simulink model "CruiseControl_Harness_SB_StandAlone"  (R2016b)
settings: Solver=FixedStepDiscrete  StartTime=0.0  StopTime=2  FixedStep=0.1  RelTol=1e-3  EnableMultiTasking=on
undefined symbols (not defined in the file): sigbuilder_block
settings Model: Creator=colosky  LastModifiedBy=colosky
settings DataIOCC: LimitDataPoints=on  SaveFormat=Array  SaveOutput=off  SignalLogging=off  DSMLogging=off  SaveTime=off
settings OptimizationCC: DefaultParameterBehavior=Inlined  InlineInvariantSignals=on  ExpressionDepthLimit=2147483647  InitFltsAndDblsToZero=on  NoFixptDivByZeroProtection=on  LifeSpan=inf
settings DebuggingCC: SignalInfNanChecking=warning  SaveWithParameterizedLinksMsg=none  UnderspecifiedInitializationDetection=Classic  MergeDetectMultiDrivingBlocksExec=none  SolverPrmCheckMsg=warning  FcnCallInpInsideContextMsg=warning  UniqueDataStoreMsg=warning  AllowSymbolicDim=off  StateNameClashWarn=warning  StrictBusMsg=ErrorOnBusTreatedAsVector  SFUnexpectedBacktrackingDiag=warning  SFNoUnconditionalDefaultTransitionDiag=warning  SFExecutionAtInitializationDiag=none
settings HardwareCC: ProdBitPerPointer=32  ProdBitPerSizeT=32  ProdBitPerPtrDiffT=32  ProdLargestAtomicFloat=None  ProdIntDivRoundTo=Undefined  ProdEndianess=Unspecified  ProdWordSize=32  ProdHWDeviceType=32-bit Generic
settings ModelReferenceCC: ModelReferenceNumInstancesAllowed=Single  PropagateSignalLabelsOutOfModel=off
settings SFSimCC: SimParseCustomCode=off
settings RTWCC: SystemTargetFile=ert.tlc  TemplateMakefile=ert_default_tmf  Description=Embedded Coder  GenerateReport=on  IncludeHyperlinkInReport=on  LaunchReport=on  PortableWordSizes=on  GenerateTraceInfo=on  GenerateTraceReport=on  GenerateTraceReportSl=on  GenerateTraceReportSf=on  GenerateTraceReportEml=on
settings CodeAppCC: IgnoreCustomStorageClasses=off  CustomSymbolStrGlobalVar=$N$M
settings ERTTargetCC: GenerateSampleERTMain=on  InlinedParameterPlacement=NonHierarchical  ERTCustomFileTemplate=example_file_process.tlc  ConvertIfToSwitch=off  SuppressUnreachableDefaultCases=off
settings ConfigComp: CovEnable=on  CovScope=ReferencedModels  CovIncludeTopModel=off  CovMetricSettings=dcme  CovHTMLOptions=-sRT=1 -sVT=0 -aTS=1 -bRG=1 -bTC=1 -hTR=0 -nFC=0 -nFD=1 -scm=1 -bcm=1 -xEv=0 -xEM=0  CovModelRefEnable=all  CovExternalEMLEnable=off  CovSFcnEnable=off  DVMode=DesignErrorDetection  DVMaxProcessTime=3000  DVDisplayUnsatisfiableObjectives=on  DVAutomaticStubbing=off  DVMakeOutputFilesUnique=off  DVParameters=on  DVParametersUseConfig=on  DVModelCoverageObjectives=MCDC  DVMaxTestCaseSteps=500  DVTestSuiteOptimization=CombinedObjectives  DVAssertions=EnableAll  DVProofAssumptions=EnableAll  DVIgnoreCovSatisfied=on  DVCoverageDataFile=CruiseControlCovManual.cvt  DVDetectIntegerOverflow=off  DVDetectDeadLogic=on  DVDetectActiveLogic=on  DVDetectFloatOverflow=off  DVMaxViolationSteps=50  DVSaveDataFile=off  DVSaveHarnessModel=on  DVHarnessModelFileName=$ModelName$_harness_SLDV  DVReportIncludeGraphics=on  PSAutoStubLUT=off

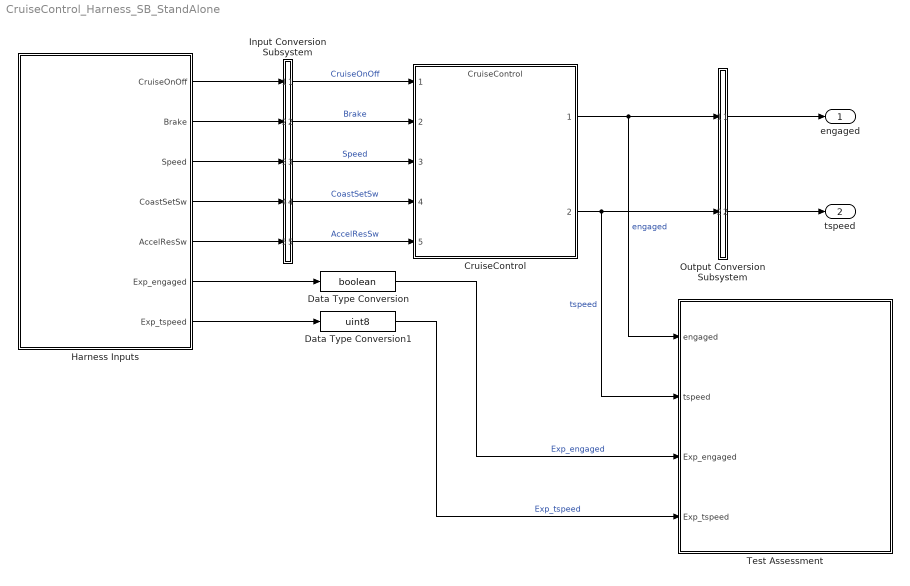
== system CruiseControl_Harness_SB_StandAlone ==
  CruiseControl : ModelReference  ModelNameDialog=CruiseControl  SimulationMode=Normal  ModelReferenceVersion=1.475
  Data Type Conversion : DataTypeConversion  OutDataTypeStr=boolean
  Data Type Conversion1 : DataTypeConversion  OutDataTypeStr=uint8
  Harness Inputs : Subsystem  Tag=STV Subsys  LoadFcn=sigbuilder_block('load',[-9.6 94.2 520.2 400.2 ]);  StartFcn=sigbuilder_block('start');  StopFcn=sigbuilder_block('stop');  ClipboardFcn=sigbuilder_block('clipboard');  mask(Sigbuilder block){tuvar=[0:10]}
      mask init:
      | if ~strcmp(get_param(bdroot(gcb),'SimulationStatus'),'stopped'),tuvar = sigbuilder_block('maskInit'); end
      settings: CopyFcn=sigbuilder_block('copy');  DeleteFcn=sigbuilder_block('delete');  ModelCloseFcn=sigbuilder_block('modelClose');  PreSaveFcn=sigbuilder_block('preSave');  PauseFcn=sigbuilder_block('pause');  ContinueFcn=sigbuilder_block('continue');  NameChangeFcn=sigbuilder_block('namechange');  OpenFcn=sigbuilder_block('open',[58.2 96 520.2 400.2 ]);  CloseFcn=sigbuilder_block('close');
      mask Display: plot(0, 0, 100, 100,[2, 2, 32, 32, 2], [68, 8, 8, 68, 68],[32, 2], [38, 38], [32, 19, 2],[53, 60, 44], [32, 17, 17, 2],[16, 16, 31, 31]);txt = getActiveGroup(gcbh);text(2, 100, txt,'verticalAlignment', 'top');
  Input Conversion Subsystem : Subsystem  Tag=_input_conv_ss_
  Output Conversion Subsystem : Subsystem  Tag=_output_conv_ss_
  Test Assessment : State Transition Table  TreatAsAtomicUnit=on
  engaged : Outport  OutDataTypeStr=boolean  PortDimensions=[1]
  tspeed : Outport  Port=2  OutDataTypeStr=uint8  PortDimensions=[1]
  wires:
  Input Conversion Subsystem/1(Out_1) -> CruiseControl/1  "CruiseOnOff"
  Input Conversion Subsystem/2(Out_2) -> CruiseControl/2  "Brake"
  Input Conversion Subsystem/3(Out_3) -> CruiseControl/3  "Speed"
  Input Conversion Subsystem/4(Out_4) -> CruiseControl/4  "CoastSetSw"
  Input Conversion Subsystem/5(Out_5) -> CruiseControl/5  "AccelResSw"
  Output Conversion Subsystem/1(Out_1) -> engaged/1
  Output Conversion Subsystem/2(Out_2) -> tspeed/1
  CruiseControl/1 -> Output Conversion Subsystem/1(In_1), Test Assessment/1(engaged)  "engaged"
  CruiseControl/2 -> Output Conversion Subsystem/2(In_2), Test Assessment/2(tspeed)  "tspeed"
  Harness Inputs/1(CruiseOnOff) -> Input Conversion Subsystem/1(In_1)
  Harness Inputs/2(Brake) -> Input Conversion Subsystem/2(In_2)
  Harness Inputs/3(Speed) -> Input Conversion Subsystem/3(In_3)
  Harness Inputs/4(CoastSetSw) -> Input Conversion Subsystem/4(In_4)
  Harness Inputs/5(AccelResSw) -> Input Conversion Subsystem/5(In_5)
  Harness Inputs/6(Exp_engaged) -> Data Type Conversion/1
  Harness Inputs/7(Exp_tspeed) -> Data Type Conversion1/1
  Data Type Conversion/1 -> Test Assessment/3(Exp_engaged)  "Exp_engaged"
  Data Type Conversion1/1 -> Test Assessment/4(Exp_tspeed)  "Exp_tspeed"

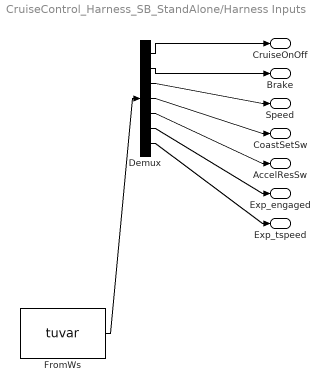
== system CruiseControl_Harness_SB_StandAlone/Harness Inputs ==
  Demux : Demux  Tag=STV Demux  Outputs=7
  FromWs : FromWorkspace  Tag=STV FromWs  VariableName=tuvar  SampleTime=0
      SigBuilderData=|
      | dataSet(1).timeRange = [0 2]
      | dataSet(1).name = 'Init Not Enable or Engaged'
      | dataSet(2).timeRange = [0 2]
      | dataSet(2).name = 'Not Engaged with Enable'
      | dataSet(3).timeRange = [0 2]
      | dataSet(3).name = 'Disengage with Disable'
      | dataSet(4).timeRange = [0 2]
      | dataSet(4).name = 'Engage 1st with CoastSetSW'
      | dataSet(5).timeRange = [0 2]
      | dataSet(5).name = 'No Engage 1st with AccelResSW'
      | dataSet(6).timeRange = [0 2]
      | dataSet(6).name = 'Disengage with Brake'
      | dataSet(7).timeRange = [0 2]
      | dataSet(7).name = 'Re-Engage with CoastSetSw'
      | dataSet(8).timeRange = [0 2]
      | dataSet(8).name = 'Re-Engage with AccelResSw'
      | dataSet(9).timeRange = [0 2]
      | dataSet(9).name = 'Engaged Decel with CoastSetSW'
      | dataSet(10).timeRange = [0 2]
      | dataSet(10).name = 'Engaged Accel with AccelResSW '
      | dataSet(11).timeRange = [0 2]
      | dataSet(11).name = 'Engagd Decel with CoastSet Hold'
      | dataSet(12).timeRange = [0 2]
      | dataSet(12).name = 'Engagd Accel with AccelRes Hold'
      | dataSet(13).timeRange = [0 2]
      | dataSet(13).name = 'Engage CoastSetSw Veh Spd'
      | dataSet(14).timeRange = [0 2]
      | dataSet(14).name = 'Engage AccelResSw Veh Spd '
      | sbobj.Name = 'Signal Builder'
      | sbobj.Groups(1).Name = 'Init Not Enable or Engaged'
      | sbobj.Groups(1).Signals(1).Name = 'CruiseOnOff'
      | sbobj.Groups(1).Signals(1).XData = [0 1 2]
      | sbobj.Groups(1).Signals(1).YData = [0 0 0]
      | sbobj.Groups(1).Signals(2).Name = 'Brake'
      | sbobj.Groups(1).Signals(2).XData = [0 1 2]
      | sbobj.Groups(1).Signals(2).YData = [0 0 0]
      | sbobj.Groups(1).Signals(3).Name = 'Speed'
      | sbobj.Groups(1).Signals(3).XData = [0 1 2]
      | sbobj.Groups(1).Signals(3).YData = [50 50 50]
      | sbobj.Groups(1).Signals(4).Name = 'CoastSetSw'
      | sbobj.Groups(1).Signals(4).XData = [0 1 2]
      | sbobj.Groups(1).Signals(4).YData = [0 0 0]
      | sbobj.Groups(1).Signals(5).Name = 'AccelResSw'
      | sbobj.Groups(1).Signals(5).XData = [0 1 2]
      | sbobj.Groups(1).Signals(5).YData = [0 0 0]
      | sbobj.Groups(1).Signals(6).Name = 'Exp_engaged'
      | sbobj.Groups(1).Signals(6).XData = [0 1 2]
      | sbobj.Groups(1).Signals(6).YData = [0 0 0]
      | sbobj.Groups(1).Signals(7).Name = 'Exp_tspeed'
      | sbobj.Groups(1).Signals(7).XData = [0 1 2]
      | sbobj.Groups(1).Signals(7).YData = [0 0 0]
      | sbobj.Groups(1).TimeRange = [0 2]
      | sbobj.Groups(2).Name = 'Not Engaged with Enable'
      | sbobj.Groups(2).Signals(1).Name = 'CruiseOnOff'
      | sbobj.Groups(2).Signals(1).XData = [0 1 1 1.5 1.5 2]
      | sbobj.Groups(2).Signals(1).YData = [0 0 1 1 0 0]
      | sbobj.Groups(2).Signals(2).Name = 'Brake'
      | sbobj.Groups(2).Signals(2).XData = [0 1 1.5 2]
      | sbobj.Groups(2).Signals(2).YData = [0 0 0 0]
      | sbobj.Groups(2).Signals(3).Name = 'Speed'
      | sbobj.Groups(2).Signals(3).XData = [0 1 1.5 2]
      | sbobj.Groups(2).Signals(3).YData = [0 0 0 0]
      | sbobj.Groups(2).Signals(4).Name = 'CoastSetSw'
      | sbobj.Groups(2).Signals(4).XData = [0 1 1.5 2]
      | sbobj.Groups(2).Signals(4).YData = [0 0 0 0]
      | sbobj.Groups(2).Signals(5).Name = 'AccelResSw'
      | sbobj.Groups(2).Signals(5).XData = [0 1 1.5 2]
      | sbobj.Groups(2).Signals(5).YData = [0 0 0 0]
      | sbobj.Groups(2).Signals(6).Name = 'Exp_engaged'
      | sbobj.Groups(2).Signals(6).XData = [0 1 1.5 2]
      | sbobj.Groups(2).Signals(6).YData = [0 0 0 0]
      | sbobj.Groups(2).Signals(7).Name = 'Exp_tspeed'
      | sbobj.Groups(2).Signals(7).XData = [0 1 1.5 2]
      | sbobj.Groups(2).Signals(7).YData = [0 0 0 0]
      | sbobj.Groups(2).TimeRange = [0 2]
      | sbobj.Groups(3).Name = 'Disengage with Disable'
      | sbobj.Groups(3).Signals(1).Name = 'CruiseOnOff'
      | sbobj.Groups(3).Signals(1).XData = [0 0.5 0.5 1 1.1 1.5 1.5 2]
      | sbobj.Groups(3).Signals(1).YData = [0 0 1 1 1 1 0 0]
      | sbobj.Groups(3).Signals(2).Name = 'Brake'
      | sbobj.Groups(3).Signals(2).XData = [0 0.5 1 1.1 1.5 2]
      | sbobj.Groups(3).Signals(2).YData = [0 0 0 0 0 0]
      | sbobj.Groups(3).Signals(3).Name = 'Speed'
      | sbobj.Groups(3).Signals(3).XData = [0 0.5 1 1.1 1.5 2]
      | sbobj.Groups(3).Signals(3).YData = [50 50 50 50 50 50]
      | sbobj.Groups(3).Signals(4).Name = 'CoastSetSw'
      | sbobj.Groups(3).Signals(4).XData = [0 0.5 1 1 1.1 1.1 1.5 2]
      | sbobj.Groups(3).Signals(4).YData = [0 0 0 1 1 0 0 0]
      | sbobj.Groups(3).Signals(5).Name = 'AccelResSw'
      | sbobj.Groups(3).Signals(5).XData = [0 0.5 1 1.1 1.5 2]
      | sbobj.Groups(3).Signals(5).YData = [0 0 0 0 0 0]
      | sbobj.Groups(3).Signals(6).Name = 'Exp_engaged'
      | sbobj.Groups(3).Signals(6).XData = [0 0.5 1 1 1.1 1.5 1.5 2]
      | sbobj.Groups(3).Signals(6).YData = [0 0 0 1 1 1 0 0]
      | sbobj.Groups(3).Signals(7).Name = 'Exp_tspeed'
      | sbobj.Groups(3).Signals(7).XData = [0 0.5 1 1 1.1 1.5 1.5 2]
      | sbobj.Groups(3).Signals(7).YData = [0 0 0 50 50 50 0 0]
      | sbobj.Groups(3).TimeRange = [0 2]
      | sbobj.Groups(4).Name = 'Engage 1st with CoastSetSW'
      | sbobj.Groups(4).Signals(1).Name = 'CruiseOnOff'
      | sbobj.Groups(4).Signals(1).XData = [0 0.5 0.5 1 1.1 2]
      | sbobj.Groups(4).Signals(1).YData = [0 0 1 1 1 1]
      | sbobj.Groups(4).Signals(2).Name = 'Brake'
      | sbobj.Groups(4).Signals(2).XData = [0 0.5 1 1.1 2]
      | sbobj.Groups(4).Signals(2).YData = [0 0 0 0 0]
      | sbobj.Groups(4).Signals(3).Name = 'Speed'
      | sbobj.Groups(4).Signals(3).XData = [0 0.5 1 1.1 2]
      | sbobj.Groups(4).Signals(3).YData = [50 50 50 50 50]
      | sbobj.Groups(4).Signals(4).Name = 'CoastSetSw'
      | sbobj.Groups(4).Signals(4).XData = [0 0.5 1 1 1.1 1.1 2]
      | sbobj.Groups(4).Signals(4).YData = [0 0 0 1 1 0 0]
      | sbobj.Groups(4).Signals(5).Name = 'AccelResSw'
      | sbobj.Groups(4).Signals(5).XData = [0 0.5 1 1.1 2]
      | sbobj.Groups(4).Signals(5).YData = [0 0 0 0 0]
      | sbobj.Groups(4).Signals(6).Name = 'Exp_engaged'
      | sbobj.Groups(4).Signals(6).XData = [0 0.5 1 1 1.1 2]
      | sbobj.Groups(4).Signals(6).YData = [0 0 0 1 1 1]
      | sbobj.Groups(4).Signals(7).Name = 'Exp_tspeed'
      | sbobj.Groups(4).Signals(7).XData = [0 0.5 1 1 1.1 2]
      | sbobj.Groups(4).Signals(7).YData = [0 0 0 50 50 50]
      | sbobj.Groups(4).TimeRange = [0 2]
      | sbobj.Groups(5).Name = 'No Engage 1st with AccelResSW'
      | sbobj.Groups(5).Signals(1).Name = 'CruiseOnOff'
      | sbobj.Groups(5).Signals(1).XData = [0 0.5 0.5 1 1.1 2]
      | sbobj.Groups(5).Signals(1).YData = [0 0 1 1 1 1]
      | sbobj.Groups(5).Signals(2).Name = 'Brake'
      | sbobj.Groups(5).Signals(2).XData = [0 0.5 1 1.1 2]
      | sbobj.Groups(5).Signals(2).YData = [0 0 0 0 0]
      | sbobj.Groups(5).Signals(3).Name = 'Speed'
      | sbobj.Groups(5).Signals(3).XData = [0 0.5 1 1.1 2]
      | sbobj.Groups(5).Signals(3).YData = [50 50 50 50 50]
      | sbobj.Groups(5).Signals(4).Name = 'CoastSetSw'
      | sbobj.Groups(5).Signals(4).XData = [0 0.5 1 1.1 2]
      | sbobj.Groups(5).Signals(4).YData = [0 0 0 0 0]
      | sbobj.Groups(5).Signals(5).Name = 'AccelResSw'
      | sbobj.Groups(5).Signals(5).XData = [0 0.5 1 1 1.1 1.1 2]
      | sbobj.Groups(5).Signals(5).YData = [0 0 0 1 1 0 0]
      | sbobj.Groups(5).Signals(6).Name = 'Exp_engaged'
      | sbobj.Groups(5).Signals(6).XData = [0 0.5 1 1.1 2]
      | sbobj.Groups(5).Signals(6).YData = [0 0 0 0 0]
      | sbobj.Groups(5).Signals(7).Name = 'Exp_tspeed'
      | sbobj.Groups(5).Signals(7).XData = [0 0.5 1 1.1 2]
      | sbobj.Groups(5).Signals(7).YData = [0 0 0 0 0]
      | sbobj.Groups(5).TimeRange = [0 2]
      | sbobj.Groups(6).Name = 'Disengage with Brake'
      | sbobj.Groups(6).Signals(1).Name = 'CruiseOnOff'
      | sbobj.Groups(6).Signals(1).XData = [0 0.5 0.5 1 1.1 1.5 1.6 2]
      | sbobj.Groups(6).Signals(1).YData = [0 0 1 1 1 1 1 1]
      | sbobj.Groups(6).Signals(2).Name = 'Brake'
      | sbobj.Groups(6).Signals(2).XData = [0 0.5 1 1.1 1.5 1.5 1.6 1.6 2]
      | sbobj.Groups(6).Signals(2).YData = [0 0 0 0 0 1 1 0 0]
      | sbobj.Groups(6).Signals(3).Name = 'Speed'
      | sbobj.Groups(6).Signals(3).XData = [0 0.5 1 1.1 1.5 1.6 2]
      | sbobj.Groups(6).Signals(3).YData = [50 50 50 50 50 50 50]
      | sbobj.Groups(6).Signals(4).Name = 'CoastSetSw'
      | sbobj.Groups(6).Signals(4).XData = [0 0.5 1 1 1.1 1.1 1.5 1.6 2]
      | sbobj.Groups(6).Signals(4).YData = [0 0 0 1 1 0 0 0 0]
      | sbobj.Groups(6).Signals(5).Name = 'AccelResSw'
      | sbobj.Groups(6).Signals(5).XData = [0 0.5 1 1.1 1.5 1.6 2]
      | sbobj.Groups(6).Signals(5).YData = [0 0 0 0 0 0 0]
      | sbobj.Groups(6).Signals(6).Name = 'Exp_engaged'
      | sbobj.Groups(6).Signals(6).XData = [0 0.5 1 1 1.1 1.5 1.5 1.6 2]
      | sbobj.Groups(6).Signals(6).YData = [0 0 0 1 1 1 0 0 0]
      | sbobj.Groups(6).Signals(7).Name = 'Exp_tspeed'
      | sbobj.Groups(6).Signals(7).XData = [0 0.5 1 1 1.1 1.5 1.6 2]
      | sbobj.Groups(6).Signals(7).YData = [0 0 0 50 50 50 50 50]
      | sbobj.Groups(6).TimeRange = [0 2]
      | sbobj.Groups(7).Name = 'Re-Engage with CoastSetSw'
      | sbobj.Groups(7).Signals(1).Name = 'CruiseOnOff'
      | sbobj.Groups(7).Signals(1).XData = [0 0.5 0.5 1 1.1 1.3 1.5 1.7 1.8 2]
      | sbobj.Groups(7).Signals(1).YData = [0 0 1 1 1 1 1 1 1 1]
      | sbobj.Groups(7).Signals(2).Name = 'Brake'
      | sbobj.Groups(7).Signals(2).XData = [0 0.5 1 1.1 1.3 1.3 1.5 1.5 1.7 1.8 2]
      | sbobj.Groups(7).Signals(2).YData = [0 0 0 0 0 1 1 0 0 0 0]
      | sbobj.Groups(7).Signals(3).Name = 'Speed'
      | sbobj.Groups(7).Signals(3).XData = [0 0.5 1 1.1 1.3 1.5 1.7 1.7 1.8 2]
      | sbobj.Groups(7).Signals(3).YData = [50 50 50 50 50 50 50 60 60 60]
      | sbobj.Groups(7).Signals(4).Name = 'CoastSetSw'
      | sbobj.Groups(7).Signals(4).XData = [0 0.5 1 1 1.1 1.1 1.3 1.5 1.7 1.7 1.8 1.8 2]
      | sbobj.Groups(7).Signals(4).YData = [0 0 0 1 1 0 0 0 0 1 1 0 0]
      | sbobj.Groups(7).Signals(5).Name = 'AccelResSw'
      | sbobj.Groups(7).Signals(5).XData = [0 0.5 1 1.1 1.3 1.5 1.7 1.8 2]
      | sbobj.Groups(7).Signals(5).YData = [0 0 0 0 0 0 0 0 0]
      | sbobj.Groups(7).Signals(6).Name = 'Exp_engaged'
      | sbobj.Groups(7).Signals(6).XData = [0 0.5 1 1 1.1 1.3 1.3 1.5 1.7 1.7 1.8 2]
      | sbobj.Groups(7).Signals(6).YData = [0 0 0 1 1 1 0 0 0 1 1 1]
      | sbobj.Groups(7).Signals(7).Name = 'Exp_tspeed'
      | sbobj.Groups(7).Signals(7).XData = [0 0.5 1 1 1.1 1.3 1.5 1.7 1.7 1.8 2]
      | sbobj.Groups(7).Signals(7).YData = [0 0 0 50 50 50 50 50 60 60 60]
      | sbobj.Groups(7).TimeRange = [0 2]
      | sbobj.Groups(8).Name = 'Re-Engage with AccelResSw'
      | sbobj.Groups(8).Signals(1).Name = 'CruiseOnOff'
      | sbobj.Groups(8).Signals(1).XData = [0 0.5 0.5 1 1.1 1.3 1.5 1.7 1.8 2]
      | sbobj.Groups(8).Signals(1).YData = [0 0 1 1 1 1 1 1 1 1]
      | sbobj.Groups(8).Signals(2).Name = 'Brake'
      | sbobj.Groups(8).Signals(2).XData = [0 0.5 1 1.1 1.3 1.3 1.5 1.5 1.7 1.8 2]
      | sbobj.Groups(8).Signals(2).YData = [0 0 0 0 0 1 1 0 0 0 0]
      | sbobj.Groups(8).Signals(3).Name = 'Speed'
      | sbobj.Groups(8).Signals(3).XData = [0 0.5 1 1.1 1.3 1.5 1.7 1.7 1.8 2]
      | sbobj.Groups(8).Signals(3).YData = [50 50 50 50 50 50 50 60 60 60]
      | sbobj.Groups(8).Signals(4).Name = 'CoastSetSw'
      | sbobj.Groups(8).Signals(4).XData = [0 0.5 1 1 1.1 1.1 1.3 1.5 1.7 1.8 2]
      | sbobj.Groups(8).Signals(4).YData = [0 0 0 1 1 0 0 0 0 0 0]
      | sbobj.Groups(8).Signals(5).Name = 'AccelResSw'
      | sbobj.Groups(8).Signals(5).XData = [0 0.5 1 1.1 1.3 1.5 1.7 1.7 1.8 1.8 2]
      | sbobj.Groups(8).Signals(5).YData = [0 0 0 0 0 0 0 1 1 0 0]
      | sbobj.Groups(8).Signals(6).Name = 'Exp_engaged'
      | sbobj.Groups(8).Signals(6).XData = [0 0.5 1 1 1.1 1.3 1.3 1.5 1.7 1.7 1.8 2]
      | sbobj.Groups(8).Signals(6).YData = [0 0 0 1 1 1 0 0 0 1 1 1]
      | sbobj.Groups(8).Signals(7).Name = 'Exp_tspeed'
      | sbobj.Groups(8).Signals(7).XData = [0 0.5 1 1 1.1 1.3 1.5 1.7 1.8 2]
      | sbobj.Groups(8).Signals(7).YData = [0 0 0 50 50 50 50 50 50 50]
      | sbobj.Groups(8).TimeRange = [0 2]
      | sbobj.Groups(9).Name = 'Engaged Decel with CoastSetSW'
      | sbobj.Groups(9).Signals(1).Name = 'CruiseOnOff'
      | sbobj.Groups(9).Signals(1).XData = [0 0.5 0.5 1 1.1 1.5 1.6 1.7 1.8 2]
      | sbobj.Groups(9).Signals(1).YData = [0 0 1 1 1 1 1 1 1 1]
      | sbobj.Groups(9).Signals(2).Name = 'Brake'
      | sbobj.Groups(9).Signals(2).XData = [0 0.5 1 1.1 1.5 1.6 1.7 1.8 2]
      | sbobj.Groups(9).Signals(2).YData = [0 0 0 0 0 0 0 0 0]
      | sbobj.Groups(9).Signals(3).Name = 'Speed'
      | sbobj.Groups(9).Signals(3).XData = [0 0.5 1 1.1 1.5 1.6 1.7 1.8 2]
      | sbobj.Groups(9).Signals(3).YData = [50 50 50 50 50 50 50 50 50]
      | sbobj.Groups(9).Signals(4).Name = 'CoastSetSw'
      | sbobj.Groups(9).Signals(4).XData = [0 0.5 1 1 1.1 1.1 1.5 1.5 1.6 1.6 1.7 1.7 1.8 1.8 2]
      | sbobj.Groups(9).Signals(4).YData = [0 0 0 1 1 0 0 1 1 0 0 1 1 0 0]
      | sbobj.Groups(9).Signals(5).Name = 'AccelResSw'
      | sbobj.Groups(9).Signals(5).XData = [0 0.5 1 1.1 1.5 1.6 1.7 1.8 2]
      | sbobj.Groups(9).Signals(5).YData = [0 0 0 0 0 0 0 0 0]
      | sbobj.Groups(9).Signals(6).Name = 'Exp_engaged'
      | sbobj.Groups(9).Signals(6).XData = [0 0.5 1 1 1.1 1.5 1.6 1.7 1.8 2]
      | sbobj.Groups(9).Signals(6).YData = [0 0 0 1 1 1 1 1 1 1]
      | sbobj.Groups(9).Signals(7).Name = 'Exp_tspeed'
      | sbobj.Groups(9).Signals(7).XData = [0 0.5 1 1 1.1 1.5 1.5 1.6 1.7 1.7 1.8 2]
      | sbobj.Groups(9).Signals(7).YData = [0 0 0 50 50 50 49 49 49 48 48 48]
      | sbobj.Groups(9).TimeRange = [0 2]
      | sbobj.Groups(10).Name = 'Engaged Accel with AccelResSW '
      | sbobj.Groups(10).Signals(1).Name = 'CruiseOnOff'
      | sbobj.Groups(10).Signals(1).XData = [0 0.5 0.5 1 1.1 1.5 1.6 1.7 1.8 2]
      | sbobj.Groups(10).Signals(1).YData = [0 0 1 1 1 1 1 1 1 1]
      | sbobj.Groups(10).Signals(2).Name = 'Brake'
      | sbobj.Groups(10).Signals(2).XData = [0 0.5 1 1.1 1.5 1.6 1.7 1.8 2]
      | sbobj.Groups(10).Signals(2).YData = [0 0 0 0 0 0 0 0 0]
      | sbobj.Groups(10).Signals(3).Name = 'Speed'
      | sbobj.Groups(10).Signals(3).XData = [0 0.5 1 1.1 1.5 1.6 1.7 1.8 2]
      | sbobj.Groups(10).Signals(3).YData = [50 50 50 50 50 50 50 50 50]
      | sbobj.Groups(10).Signals(4).Name = 'CoastSetSw'
      | sbobj.Groups(10).Signals(4).XData = [0 0.5 1 1 1.1 1.1 1.5 1.6 1.7 1.8 2]
      | sbobj.Groups(10).Signals(4).YData = [0 0 0 1 1 0 0 0 0 0 0]
      | sbobj.Groups(10).Signals(5).Name = 'AccelResSw'
      | sbobj.Groups(10).Signals(5).XData = [0 0.5 1 1.1 1.5 1.5 1.6 1.6 1.7 1.7 1.8 1.8 2]
      | sbobj.Groups(10).Signals(5).YData = [0 0 0 0 0 1 1 0 0 1 1 0 0]
      | sbobj.Groups(10).Signals(6).Name = 'Exp_engaged'
      | sbobj.Groups(10).Signals(6).XData = [0 0.5 1 1 1.1 1.5 1.6 1.7 1.8 2]
      | sbobj.Groups(10).Signals(6).YData = [0 0 0 1 1 1 1 1 1 1]
      | sbobj.Groups(10).Signals(7).Name = 'Exp_tspeed'
      | sbobj.Groups(10).Signals(7).XData = [0 0.5 1 1 1.1 1.5 1.5 1.6 1.7 1.7 1.8 2]
      | sbobj.Groups(10).Signals(7).YData = [0 0 0 50 50 50 51 51 51 52 52 52]
      | sbobj.Groups(10).TimeRange = [0 2]
      | sbobj.Groups(11).Name = 'Engagd Decel with CoastSet Hold'
      | sbobj.Groups(11).Signals(1).Name = 'CruiseOnOff'
      | sbobj.Groups(11).Signals(1).XData = [0 0.2 0.2 0.5 0.6 1 1.1 1.3 1.5 1.7 1.8 2]
      | sbobj.Groups(11).Signals(1).YData = [0 0 1 1 1 1 1 1 1 1 1 1]
      | sbobj.Groups(11).Signals(2).Name = 'Brake'
      | sbobj.Groups(11).Signals(2).XData = [0 0.2 0.5 0.6 1 1.1 1.3 1.5 1.7 1.8 2]
      | sbobj.Groups(11).Signals(2).YData = [0 0 0 0 0 0 0 0 0 0 0]
      | sbobj.Groups(11).Signals(3).Name = 'Speed'
      | sbobj.Groups(11).Signals(3).XData = [0 0.2 0.5 0.6 0.6 1 1.1 1.3 1.5 1.7 1.8 2]
      | sbobj.Groups(11).Signals(3).YData = [50 50 50 50 40 40 40 40 40 40 40 40]
      | sbobj.Groups(11).Signals(4).Name = 'CoastSetSw'
      | sbobj.Groups(11).Signals(4).XData = [0 0.2 0.5 0.5 0.6 0.6 1 1 1.1 1.1 1.3 1.3 1.5 1.7 1.8 1.8 2]
      | sbobj.Groups(11).Signals(4).YData = [0 0 0 1 1 0 0 1 1 0 0 1 1 1 1 0 0]
      | sbobj.Groups(11).Signals(5).Name = 'AccelResSw'
      | sbobj.Groups(11).Signals(5).XData = [0 0.2 0.5 0.6 1 1.1 1.3 1.5 1.7 1.8 2]
      | sbobj.Groups(11).Signals(5).YData = [0 0 0 0 0 0 0 0 0 0 0]
      | sbobj.Groups(11).Signals(6).Name = 'Exp_engaged'
      | sbobj.Groups(11).Signals(6).XData = [0 0.2 0.5 0.5 0.6 1 1.1 1.3 1.5 1.7 1.8 2]
      | sbobj.Groups(11).Signals(6).YData = [0 0 0 1 1 1 1 1 1 1 1 1]
      | sbobj.Groups(11).Signals(7).Name = 'Exp_tspeed'
      | sbobj.Groups(11).Signals(7).XData = [0 0.2 0.5 0.5 0.6 1 1 1.1 1.3 1.3 1.5 1.5 1.7 1.7 1.8 2]
      | sbobj.Groups(11).Signals(7).YData = [0 0 0 50 50 50 49 49 49 48 48 47 47 46 46 46]
      | sbobj.Groups(11).TimeRange = [0 2]
      | sbobj.Groups(12).Name = 'Engagd Accel with AccelRes Hold'
      | sbobj.Groups(12).Signals(1).Name = 'CruiseOnOff'
      | sbobj.Groups(12).Signals(1).XData = [0 0.2 0.2 0.5 0.6 1 1.1 1.3 1.5 1.7 1.8 2]
      | sbobj.Groups(12).Signals(1).YData = [0 0 1 1 1 1 1 1 1 1 1 1]
      | sbobj.Groups(12).Signals(2).Name = 'Brake'
      | sbobj.Groups(12).Signals(2).XData = [0 0.2 0.5 0.6 1 1.1 1.3 1.5 1.7 1.8 2]
      | sbobj.Groups(12).Signals(2).YData = [0 0 0 0 0 0 0 0 0 0 0]
      | sbobj.Groups(12).Signals(3).Name = 'Speed'
      | sbobj.Groups(12).Signals(3).XData = [0 0.2 0.5 0.6 0.6 1 1.1 1.3 1.5 1.7 1.8 2]
      | sbobj.Groups(12).Signals(3).YData = [50 50 50 50 40 40 40 40 40 40 40 40]
      | sbobj.Groups(12).Signals(4).Name = 'CoastSetSw'
      | sbobj.Groups(12).Signals(4).XData = [0 0.2 0.5 0.5 0.6 0.6 1 1.1 1.3 1.5 1.7 1.8 2]
      | sbobj.Groups(12).Signals(4).YData = [0 0 0 1 1 0 0 0 0 0 0 0 0]
      | sbobj.Groups(12).Signals(5).Name = 'AccelResSw'
      | sbobj.Groups(12).Signals(5).XData = [0 0.2 0.5 0.6 1 1 1.1 1.1 1.3 1.3 1.5 1.7 1.8 1.8 2]
      | sbobj.Groups(12).Signals(5).YData = [0 0 0 0 0 1 1 0 0 1 1 1 1 0 0]
      | sbobj.Groups(12).Signals(6).Name = 'Exp_engaged'
      | sbobj.Groups(12).Signals(6).XData = [0 0.2 0.5 0.5 0.6 1 1.1 1.3 1.5 1.7 1.8 2]
      | sbobj.Groups(12).Signals(6).YData = [0 0 0 1 1 1 1 1 1 1 1 1]
      | sbobj.Groups(12).Signals(7).Name = 'Exp_tspeed'
      | sbobj.Groups(12).Signals(7).XData = [0 0.2 0.5 0.5 0.6 1 1 1.1 1.3 1.3 1.5 1.5 1.7 1.7 1.8 2]
      | sbobj.Groups(12).Signals(7).YData = [0 0 0 50 50 50 51 51 51 52 52 53 53 54 54 54]
      | sbobj.Groups(12).TimeRange = [0 2]
      | sbobj.Groups(13).Name = 'Engage CoastSetSw Veh Spd'
      | sbobj.Groups(13).Signals(1).Name = 'CruiseOnOff'
      | sbobj.Groups(13).Signals(1).XData = [0 0.5 0.5 1 1.1 1.3 1.5 1.7 1.8 2]
      | sbobj.Groups(13).Signals(1).YData = [0 0 1 1 1 1 1 1 1 1]
      | sbobj.Groups(13).Signals(2).Name = 'Brake'
      | sbobj.Groups(13).Signals(2).XData = [0 0.5 1 1.1 1.3 1.5 1.7 1.8 2]
      | sbobj.Groups(13).Signals(2).YData = [0 0 0 0 0 0 0 0 0]
      | sbobj.Groups(13).Signals(3).Name = 'Speed'
      | sbobj.Groups(13).Signals(3).XData = [0 0.5 1 1.1 1.3 1.3 1.5 1.7 1.7 1.8 2]
      | sbobj.Groups(13).Signals(3).YData = [19 19 19 19 19 91 91 91 60 60 60]
      | sbobj.Groups(13).Signals(4).Name = 'CoastSetSw'
      | sbobj.Groups(13).Signals(4).XData = [0 0.5 1 1 1.1 1.1 1.3 1.3 1.5 1.5 1.7 1.7 1.8 1.8 2]
      | sbobj.Groups(13).Signals(4).YData = [0 0 0 1 1 0 0 1 1 0 0 1 1 0 0]
      | sbobj.Groups(13).Signals(5).Name = 'AccelResSw'
      | sbobj.Groups(13).Signals(5).XData = [0 0.5 1 1.1 1.3 1.5 1.7 1.8 2]
      | sbobj.Groups(13).Signals(5).YData = [0 0 0 0 0 0 0 0 0]
      | sbobj.Groups(13).Signals(6).Name = 'Exp_engaged'
      | sbobj.Groups(13).Signals(6).XData = [0 0.5 1 1.1 1.3 1.5 1.7 1.7 1.8 2]
      | sbobj.Groups(13).Signals(6).YData = [0 0 0 0 0 0 0 1 1 1]
      | sbobj.Groups(13).Signals(7).Name = 'Exp_tspeed'
      | sbobj.Groups(13).Signals(7).XData = [0 0.5 1 1.1 1.3 1.5 1.7 1.7 1.8 2]
      | sbobj.Groups(13).Signals(7).YData = [0 0 0 0 0 0 0 60 60 60]
      | sbobj.Groups(13).TimeRange = [0 2]
      | sbobj.Groups(14).Name = 'Engage AccelResSw Veh Spd '
      | sbobj.Groups(14).Signals(1).Name = 'CruiseOnOff'
      | sbobj.Groups(14).Signals(1).XData = [0 0.5 0.5 0.7 0.8 0.9 1 1.1 1.2 1.3 1.4 1.6 1.7 2]
      | sbobj.Groups(14).Signals(1).YData = [0 0 1 1 1 1 1 1 1 1 1 1 1 1]
      | sbobj.Groups(14).Signals(2).Name = 'Brake'
      | sbobj.Groups(14).Signals(2).XData = [0 0.5 0.7 0.8 0.9 0.9 1 1 1.1 1.2 1.3 1.4 1.6 1.7 2]
      | sbobj.Groups(14).Signals(2).YData = [0 0 0 0 0 1 1 0 0 0 0 0 0 0 0]
      | sbobj.Groups(14).Signals(3).Name = 'Speed'
      | sbobj.Groups(14).Signals(3).XData = [0 0.5 0.7 0.8 0.9 1 1.1 1.1 1.2 1.3 1.3 1.4 1.6 1.6 1.7 2]
      | sbobj.Groups(14).Signals(3).YData = [50 50 50 50 50 50 50 19 19 19 91 91 91 60 60 60]
      | sbobj.Groups(14).Signals(4).Name = 'CoastSetSw'
      | sbobj.Groups(14).Signals(4).XData = [0 0.5 0.7 0.7 0.8 0.8 0.9 1 1.1 1.2 1.3 1.4 1.6 1.7 2]
      | sbobj.Groups(14).Signals(4).YData = [0 0 0 1 1 0 0 0 0 0 0 0 0 0 0]
      | sbobj.Groups(14).Signals(5).Name = 'AccelResSw'
      | sbobj.Groups(14).Signals(5).XData = [0 0.5 0.7 0.8 0.9 1 1.1 1.1 1.2 1.2 1.3 1.3 1.4 1.4 1.6 1.6 1.7 1.7 2]
      | sbobj.Groups(14).Signals(5).YData = [0 0 0 0 0 0 0 1 1 0 0 1 1 0 0 1 1 0 0]
      | sbobj.Groups(14).Signals(6).Name = 'Exp_engaged'
      | sbobj.Groups(14).Signals(6).XData = [0 0.5 0.7 0.7 0.8 0.9 0.9 1 1.1 1.2 1.3 1.4 1.6 1.6 1.7 2]
      | sbobj.Groups(14).Signals(6).YData = [0 0 0 1 1 1 0 0 0 0 0 0 0 1 1 1]
      | sbobj.Groups(14).Signals(7).Name = 'Exp_tspeed'
      | sbobj.Groups(14).Signals(7).XData = [0 0.5 0.7 0.7 0.8 0.9 1 1.1 1.2 1.3 1.4 1.6 1.7 2]
      | sbobj.Groups(14).Signals(7).YData = [0 0 0 50 50 50 50 50 50 50 50 50 50 50]
      | sbobj.Groups(14).TimeRange = [0 2]
  CruiseOnOff : Outport
  Brake : Outport  Tag=STV Outport  Port=2
  Speed : Outport  Tag=STV Outport  Port=3
  CoastSetSw : Outport  Tag=STV Outport  Port=4
  AccelResSw : Outport  Tag=STV Outport  Port=5
  Exp_engaged : Outport  Tag=STV Outport  Port=6
  Exp_tspeed : Outport  Tag=STV Outport  Port=7
  wires:
  FromWs/1 -> Demux/1
  Demux/1 -> CruiseOnOff/1
  Demux/2 -> Brake/1
  Demux/3 -> Speed/1
  Demux/4 -> CoastSetSw/1
  Demux/5 -> AccelResSw/1
  Demux/6 -> Exp_engaged/1
  Demux/7 -> Exp_tspeed/1

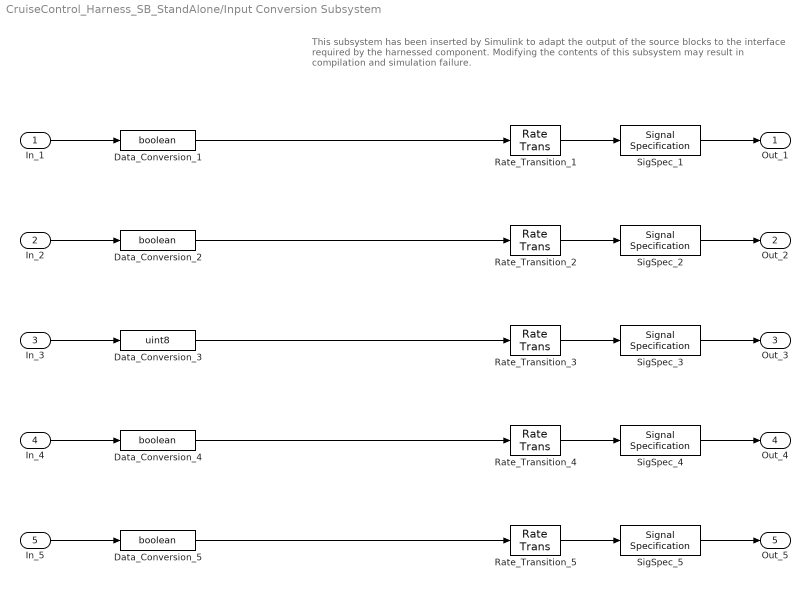
== system CruiseControl_Harness_SB_StandAlone/Input Conversion Subsystem ==
  note: This subsystem has been inserted by Simulink to adapt the output of the source blocks to the interface required by the harnessed component.
      |  Modifying the contents of this subsystem may result in compilation and simulation failure.
  In_1 : Inport
  In_2 : Inport  Port=2
  In_3 : Inport  Port=3
  In_4 : Inport  Port=4
  In_5 : Inport  Port=5
  Data_Conversion_{1..2,4..5} (4 alike) : DataTypeConversion  OutDataTypeStr=boolean  SaturateOnIntegerOverflow=on  RndMeth=Zero
  Data_Conversion_3 : DataTypeConversion  OutDataTypeStr=uint8  SaturateOnIntegerOverflow=on  RndMeth=Zero
  Rate_Transition_{1..5} (5 alike) : RateTransition  OutPortSampleTime=0.1
  SigSpec_{1..2,4..5} (4 alike) : SignalSpecification  OutDataTypeStr=boolean  Dimensions=[1]  SampleTime=0.1
  SigSpec_3 : SignalSpecification  OutDataTypeStr=uint8  Dimensions=[1]  SampleTime=0.1
  Out_1 : Outport
  Out_2 : Outport  Port=2
  Out_3 : Outport  Port=3
  Out_4 : Outport  Port=4
  Out_5 : Outport  Port=5
  wires:
  SigSpec_5/1 -> Out_5/1
  SigSpec_4/1 -> Out_4/1
  SigSpec_3/1 -> Out_3/1
  SigSpec_2/1 -> Out_2/1
  SigSpec_1/1 -> Out_1/1
  Rate_Transition_5/1 -> SigSpec_5/1
  Rate_Transition_4/1 -> SigSpec_4/1
  Rate_Transition_3/1 -> SigSpec_3/1
  Rate_Transition_2/1 -> SigSpec_2/1
  Rate_Transition_1/1 -> SigSpec_1/1
  Data_Conversion_5/1 -> Rate_Transition_5/1
  In_5/1 -> Data_Conversion_5/1
  Data_Conversion_4/1 -> Rate_Transition_4/1
  In_4/1 -> Data_Conversion_4/1
  Data_Conversion_3/1 -> Rate_Transition_3/1
  In_3/1 -> Data_Conversion_3/1
  Data_Conversion_2/1 -> Rate_Transition_2/1
  In_2/1 -> Data_Conversion_2/1
  Data_Conversion_1/1 -> Rate_Transition_1/1
  In_1/1 -> Data_Conversion_1/1

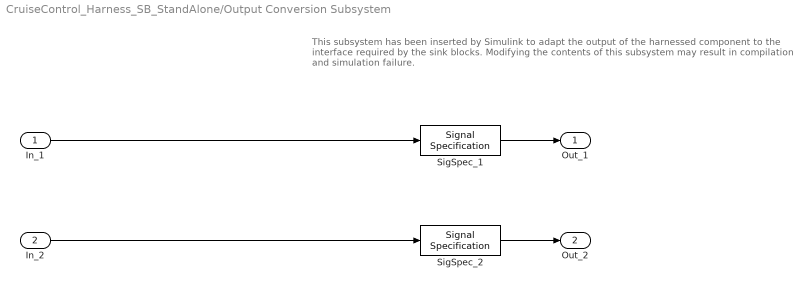
== system CruiseControl_Harness_SB_StandAlone/Output Conversion Subsystem ==
  note: This subsystem has been inserted by Simulink to adapt the output of the harnessed component to the interface required by the sink blocks.
      |  Modifying the contents of this subsystem may result in compilation and simulation failure.
  In_1 : Inport
  In_2 : Inport  Port=2
  SigSpec_1 : SignalSpecification  OutDataTypeStr=boolean  Dimensions=[1]  SampleTime=0.1
  SigSpec_2 : SignalSpecification  OutDataTypeStr=uint8  Dimensions=[1]  SampleTime=0.1
  Out_1 : Outport
  Out_2 : Outport  Port=2
  wires:
  In_2/1 -> SigSpec_2/1
  In_1/1 -> SigSpec_1/1
  SigSpec_2/1 -> Out_2/1
  SigSpec_1/1 -> Out_1/1

== stateflow chart CruiseControl_Harness_SB_StandAlone/Test Assessment ==
  settings: stateMachineType=SIMPLIFIED_MACHINE
  state Assessment
    verify(engaged==Exp_engaged,'engaged:eq:Exp_engaged','Failed output check for "engaged"');
    verify(tspeed==Exp_tspeed,'tspeed:eq:Exp_tspeed','Failed output check for "tspeed"');
  (default) -> Assessment
  data: engaged input boolean size=[1]; tspeed input uint8 size=[1]; Exp_engaged input; Exp_tspeed input
